simulink model "h175_model_stack_harness"  (R2023a)
settings: Solver=VariableStepAuto  StartTime=0.0  StopTime=4750  MaxStep=50  RelTol=1e-2
undefined symbols (not defined in the file): N2_T, sigbuilder_block
libraries: fl_lib x13, nesl_utility x11, SimscapeFluids_lib x2
(part 1 of 3)
settings Model: Creator=adrian.taveras  LastModifiedBy=stefan.notter
settings SolverCC: MaxConsecutiveMinStep=10  DecoupledContinuousIntegration=on
settings SimscapeCC: SimscapeLogType=all

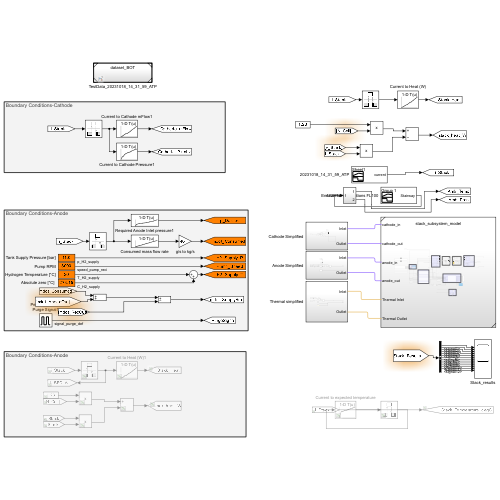
[thumbnail: Simulink's stored preview of the top-level diagram]
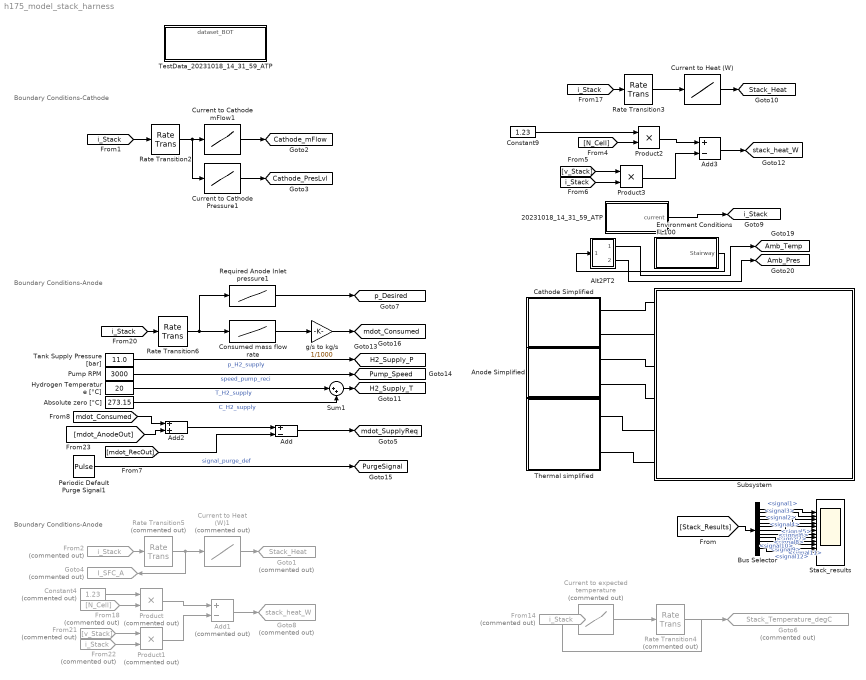
== system h175_model_stack_harness ==
  note: Boundary Conditions-Cathode
  note: Boundary Conditions-Anode
  note: Boundary Conditions-Anode
  20231018_14_31_59_ATP : Subsystem  Tag=STV Subsys  LoadFcn=sigbuilder_block('load');  StartFcn=sigbuilder_block('start');  StopFcn=sigbuilder_block('stop');  ClipboardFcn=sigbuilder_block('clipboard');  mask(Sigbuilder block){tuvar=[0:10]}
      mask help: Simulink:masks:SigbuilderBlock_MD
      mask init:
      | if ~strcmp(get_param(bdroot(gcbh),'SimulationStatus'),'stopped') tuvar = sigbuilder_block('maskInit'); end
      settings: CopyFcn=sigbuilder_block('copy');  DeleteFcn=sigbuilder_block('delete');  ModelCloseFcn=sigbuilder_block('modelClose');  PreSaveFcn=sigbuilder_block('preSave');  PauseFcn=sigbuilder_block('pause');  ContinueFcn=sigbuilder_block('continue');  NameChangeFcn=sigbuilder_block('namechange');  OpenFcn=sigbuilder_block('open',[725.25 330.75 938.25 556.5 ]);  CloseFcn=sigbuilder_block('close');
      mask Display: plot(0, 0, 100, 100,[2, 2, 32, 32, 2], [68, 8, 8, 68, 68],[32, 2], [38, 38], [32, 19, 2],[53, 60, 44], [32, 17, 17, 2],[16, 16, 31, 31]);txt = getActiveGroup(gcbh);text(2, 100, txt,'verticalAlignment', 'top');
  "Absolute zero [°C] " : Constant  Value=273.15
  Add : Sum  Inputs=+-
  Add1 : Sum  Commented=on  Inputs=+-
  Add2 : Sum
  Add3 : Sum  Inputs=+-
  Alt2PT2 : Subsystem
  Anode Simplified : Subsystem
  Bus Selector : BusSelector  OutputSignals=signal1,signal2,signal3,signal4,signal5,signal6,signal7,signal8,signal9,signal10,signal11,signal12
  Cathode Simplified : Subsystem
  Constant4 : Constant  Commented=on  Value=1.23
  Constant9 : Constant  Value=1.23
  Consumed mass flow rate : Lookup_n-D  NumberOfTableDimensions=1  BreakpointsForDimension1=[0;20;100;200;300;400;500;600]  Table=[0;0.1;0.5;1;1.5;2;2.5;3]  InternalRulePriority=Speed  RndMeth=Simplest
  Current to Cathode Pressure1 : Lookup_n-D  NumberOfTableDimensions=1  BreakpointsForDimension1=[0;50;100;150;200;250;300;350;400;510;600]  Table=[101330;140000;150000;175000;185000;195000;202500;210000;220000;235000;250000]  InternalRulePriority=Speed  RndMeth=Simplest
  Current to Cathode mFlow1 : Lookup_n-D  NumberOfTableDimensions=1  BreakpointsForDimension1=[0;50;100;150;200;250;300;350;400;510;600]  Table=[0;0.01;0.0225;0.035;0.045;0.055;0.068;0.0825;0.1;0.135;0.167]  InternalRulePriority=Speed  RndMeth=Simplest
  Current to Heat (W) : Lookup_n-D  NumberOfTableDimensions=1  BreakpointsForDimension1=[0:50:400]  Table=[0, 9932, 21438, 33442,47123, 59491, 77033, 93585, 112042]  InternalRulePriority=Speed  RndMeth=Simplest
  Current to Heat (W)1 : Lookup_n-D  Commented=on  NumberOfTableDimensions=1  BreakpointsForDimension1=[0:50:400]  Table=[0, 9932, 21438, 33442,47123, 59491, 77033, 93585, 112042]  InternalRulePriority=Speed  RndMeth=Simplest
  Current to expected temperature : Lookup_n-D  Commented=on  NumberOfTableDimensions=1  BreakpointsForDimension1=[0 50 100 150 200 250 300 350 400]  Table=[60 78 80 82 84 86 88 90 93]  InternalRulePriority=Speed  RndMeth=Simplest
  Environment Conditions FL100 : Subsystem  Tag=STV Subsys  LoadFcn=sigbuilder_block('load');  StartFcn=sigbuilder_block('start');  StopFcn=sigbuilder_block('stop');  ClipboardFcn=sigbuilder_block('clipboard');  mask(Sigbuilder block){tuvar=[0:10]}
      mask help: Simulink:masks:SigbuilderBlock_MD
      mask init:
      | if ~strcmp(get_param(bdroot(gcbh),'SimulationStatus'),'stopped') tuvar = sigbuilder_block('maskInit'); end
      settings: CopyFcn=sigbuilder_block('copy');  DeleteFcn=sigbuilder_block('delete');  ModelCloseFcn=sigbuilder_block('modelClose');  PreSaveFcn=sigbuilder_block('preSave');  PauseFcn=sigbuilder_block('pause');  ContinueFcn=sigbuilder_block('continue');  NameChangeFcn=sigbuilder_block('namechange');  OpenFcn=sigbuilder_block('open',[6 30 1908 951.75 ]);  CloseFcn=sigbuilder_block('close');
      mask Display: plot(0, 0, 100, 100,[2, 2, 32, 32, 2], [68, 8, 8, 68, 68],[32, 2], [38, 38], [32, 19, 2],[53, 60, 44], [32, 17, 17, 2],[16, 16, 31, 31]);txt = getActiveGroup(gcbh);text(2, 100, txt,'verticalAlignment', 'top');
  From14 : From  Commented=on  GotoTag=i_Stack  TagVisibility=global
  From18 : From  Commented=on  GotoTag=N_Cell
  From2 : From  Commented=on  GotoTag=i_Stack  TagVisibility=global
  From21 : From  Commented=on  GotoTag=v_Stack  TagVisibility=global
  From22 : From  Commented=on  GotoTag=i_Stack  TagVisibility=global
  Goto1 : Goto  Commented=on  GotoTag=Stack_Heat  TagVisibility=global
  Goto4 : Goto  Commented=on  GotoTag=I_SFC_A  TagVisibility=global
  Goto6 : Goto  Commented=on  GotoTag=Stack_Temperature_degC  TagVisibility=global
  Goto8 : Goto  Commented=on  GotoTag=stack_heat_W  TagVisibility=global
  Hydrogen Temperature [°C] : Constant  Value=20
  Periodic Default Purge Signal1 : DiscretePulseGenerator  PulseType=Time based  Period=3  PulseWidth=5
  Product : Product  Commented=on
  Product1 : Product  Commented=on
  Product2 : Product
  Product3 : Product
  Pump RPM : Constant  Value=3000
  Rate Transition2 : RateTransition
  Rate Transition3 : RateTransition
  Rate Transition4 : RateTransition  Commented=on
  Rate Transition5 : RateTransition  Commented=on
  Rate Transition6 : RateTransition
  Required Anode Inlet pressure1 : Lookup_n-D  NumberOfTableDimensions=1  BreakpointsForDimension1=[0;20;100;200;300;400;500;600]  Table=[1;1.4;1.6;1.7;1.8;2;2.3;2.6]  InternalRulePriority=Speed  RndMeth=Simplest
  Stack_results : Scope  NumInputPorts=12
  Subsystem : Subsystem  InitFcn=|  ReferencedSubsystem=stack_subsystem_model
      | addpath(genpath('p10_doe_files/'))
      | run('stack_subsystem_parameters.m')
      | run('stack_subsystem_supply_bus_definitions.m')
      settings: PortSchema="{\"entries\":[{\"content\":{\"sides\":[{\"content\":{\"connectorIds\":[\"RConn1\",\"RConn2\",\"LConn1\",\"LConn2\",\"LConn3\",\"LConn4\"]},\"type\":\"ConnectorPlacement.EquallySpacedRectSide\",\"uuid\":\"f7417d0d-e48e-4edc-84f7-16cb6b1fd341\"},{\"content\":{\"side\":\"RIGHT\"},\"type\":\"ConnectorPlacement.EquallySpacedRectSide\",\"uuid\":\"dd727874-0c87-4720-9a58-e9e43c2cfc5b\"},{\"content\":{\"side\":\"TOP\"},\"type\":\"ConnectorPlacement.EquallySpacedRectSide\",\"uuid\":\"042cb514-9034-4c64-aaa6-55fccd9e3c82\"},{\"content\":{\"side\":\"BOTTOM\"},\"type\":\"ConnectorPlacement.EquallySpacedRectSide\",\"uuid\":\"dba865e7-7c98-4866-84bd-6f3d01b8a3bd\"}]},\"type\":\"ConnectorPlacement.EquallySpacedConnector\",\"uuid\":\"b4ac4c8a-745a-415f-9259-8b2ea3c16805\"}],\"packageUris\":[\"http://schema.mathworks.com/mf0/Connector/R2020b\"],\"version\":\"1.0\"}"
  Sum1 : Sum  Inputs=|++
  Tank Supply Pressure [bar] : Constant  Value=11.0
  TestData_20231018_14_31_59_ATP : ModelReference  ModelNameDialog=dataset_BOT.slx  SimulationMode=Normal  ModelReferenceVersion=1.3
  Thermal simplified : Subsystem
  g/s to kg/s : Gain  Gain=1/1000
  tag scope: Amb_Pres=global, Amb_Temp=global, Cathode_PresLvl=global, Cathode_mFlow=global, H2_Supply_P=global, H2_Supply_T=global, Pump_Speed=global, PurgeSignal=global, Stack_Heat=global, i_Stack=global, mdot_Consumed=global, mdot_SupplyReq=global, p_Desired=global, stack_heat_W=global
  wires:
  [mdot_RecOut] -> Add/2
  [mdot_AnodeOut] -> Add2/2
  Add2/1 -> Add/1
  Product1/1 -> Add1/2
  Rate Transition4/1 -> Current to expected temperature/1
  Required Anode Inlet pressure1/1 -> [p_Desired]
  [i_Stack] -> Rate Transition2/1
  From14/1 -> Rate Transition4/1
  Current to Cathode Pressure1/1 -> [Cathode_PresLvl]
  Constant4/1 -> Product/1
  [mdot_Consumed] -> Add2/1
  Periodic Default Purge Signal1/1 -> [PurgeSignal]  "signal_purge_def"
  From18/1 -> Product/2
  Product/1 -> Add1/1
  Add1/1 -> Goto8/1
  From22/1 -> Product1/2
  Current to Heat (W)1/1 -> Goto1/1
  Current to Cathode mFlow1/1 -> [Cathode_mFlow]
  [i_Stack] -> Rate Transition6/1
  From2/1 -> Rate Transition5/1
  Current to expected temperature/1 -> Goto6/1
  Rate Transition6/1 -> Required Anode Inlet pressure1/1, Consumed mass flow rate/1
  Rate Transition2/1 -> Current to Cathode Pressure1/1, Current to Cathode mFlow1/1
  Rate Transition5/1 -> Goto4/1, Current to Heat (W)1/1
  Tank Supply Pressure [bar]/1 -> [H2_Supply_P]  "p_H2_supply"
  Pump RPM/1 -> [Pump_Speed]  "speed_pump_reci"
  From21/1 -> Product1/1
  Add/1 -> [mdot_SupplyReq]
  Hydrogen Temperature [°C]/1 -> Sum1/1  "T_H2_supply"
  "Absolute zero [°C] "/1 -> Sum1/2  "C_H2_supply"
  g/s to kg/s/1 -> [mdot_Consumed]
  Sum1/1 -> [H2_Supply_T]
  Consumed mass flow rate/1 -> g/s to kg/s/1
  Alt2PT2/2(Out2) -> [Amb_Pres]
  Environment Conditions FL100/1(Stairway) -> Alt2PT2/1(In1)
  Alt2PT2/1(Out1) -> [Amb_Temp]
  Product3/1 -> Add3/2
  [v_Stack] -> Product3/1
  Constant9/1 -> Product2/1
  Product2/1 -> Add3/1
  [i_Stack] -> Product3/2
  Add3/1 -> [stack_heat_W]
  Current to Heat (W)/1 -> [Stack_Heat]
  [i_Stack] -> Rate Transition3/1
  Rate Transition3/1 -> Current to Heat (W)/1
  [N_Cell] -> Product2/2
  20231018_14_31_59_ATP/1(current) -> [i_Stack]
  [Stack_Results] -> Bus Selector/1
  Bus Selector/1 -> Stack_results/1  "<signal1>"
  Bus Selector/2 -> Stack_results/2  "<signal2>"
  Bus Selector/3 -> Stack_results/3  "<signal3>"
  Bus Selector/4 -> Stack_results/4  "<signal4>"
  Bus Selector/5 -> Stack_results/5  "<signal5>"
  Bus Selector/6 -> Stack_results/6  "<signal6>"
  Bus Selector/7 -> Stack_results/7  "<signal7>"
  Bus Selector/8 -> Stack_results/8  "<signal8>"
  Bus Selector/9 -> Stack_results/10  "<signal9>"
  Bus Selector/10 -> Stack_results/9  "<signal10>"
  Bus Selector/11 -> Stack_results/11  "<signal11>"
  Bus Selector/12 -> Stack_results/12  "<signal12>"
  connections:
  Thermal simplified/RConn1 -- Subsystem/LConn3
  Subsystem/LConn4 -- Thermal simplified/RConn2
  Anode Simplified/RConn1 -- Subsystem/LConn1
  Anode Simplified/RConn2 -- Subsystem/LConn2
  Cathode Simplified/RConn1 -- Subsystem/RConn1
  Cathode Simplified/RConn2 -- Subsystem/RConn2

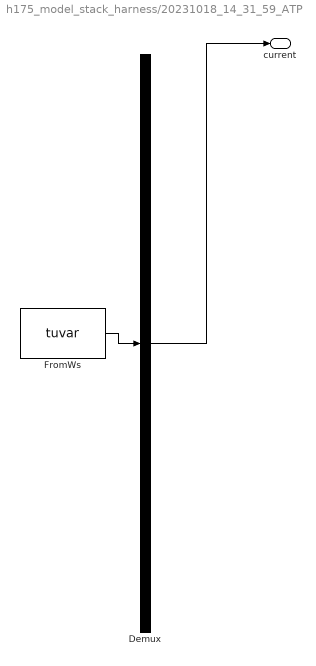
== system h175_model_stack_harness/20231018_14_31_59_ATP ==
  Demux : Demux  Tag=STV Demux  Outputs=1
      settings: DisplayOption=none
  FromWs : FromWorkspace  Tag=STV FromWs  VariableName=tuvar
      SigBuilderData=|
      | common.afterFinalStr = 'Extrapolate'
      | common.sampleTime = 0
      | dataSet.timeRange = [0 4735]
      | dataSet.name = 'Sheet1'
      | sbobj.Groups.Name = 'Sheet1'
      | sbobj.Groups.Signals.Name = 'current'
      | sbobj.Groups.Signals.XData = [0 710 730 830 850 1000 1020 1080 1100 1200 1230 1260 1270 1320 1340 1390 1405 1455 1475 1525 1565 3990 4000 4030 4090 4130 4245 4270 4345 4355 4385 4395 4735]
      | sbobj.Groups.Signals.YData = [5 5 45 45 100 100 200 200 300 300 45 45 50 50 200 200 300 300 100 100 420 420 340 420 260 340 340 50 50 45 45 5 5]
      | sbobj.Groups.TimeRange = [0 4735]
  current : Outport  Tag=STV Outport
  wires:
  Demux/1 -> current/1
  FromWs/1 -> Demux/1

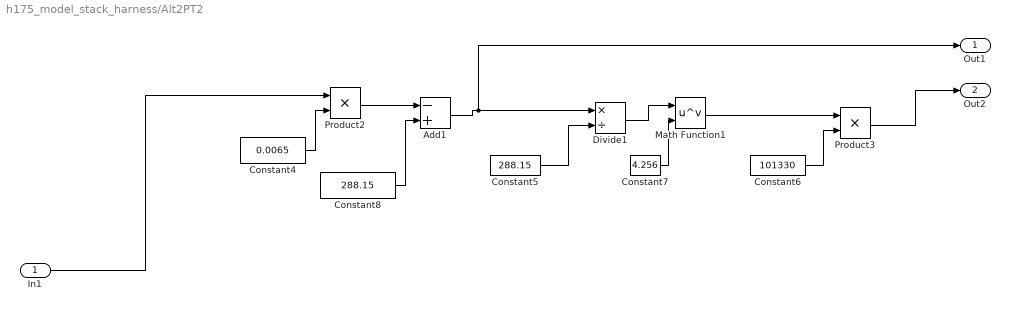
== system h175_model_stack_harness/Alt2PT2 ==
  In1 : Inport
  Add1 : Sum  Inputs=-+
  Constant4 : Constant  Value=0.0065
  Constant5 : Constant  Value=288.15
  Constant6 : Constant  Value=101330
  Constant7 : Constant  Value=4.256
  Constant8 : Constant  Value=288.15
  Divide1 : Product  Inputs=*/
  Math Function1 : Math  Operator=pow
  Product2 : Product
  Product3 : Product
  Out1 : Outport
  Out2 : Outport  Port=2
  wires:
  Constant5/1 -> Divide1/2
  Constant8/1 -> Add1/2
  In1/1 -> Product2/1
  Add1/1 -> Out1/1, Divide1/1
  Constant4/1 -> Product2/2
  Math Function1/1 -> Product3/1
  Constant7/1 -> Math Function1/2
  Divide1/1 -> Math Function1/1
  Product2/1 -> Add1/1
  Constant6/1 -> Product3/2
  Product3/1 -> Out2/1

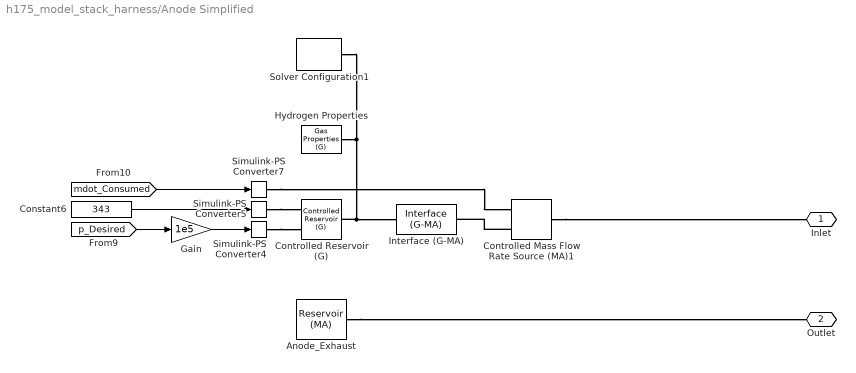
== system h175_model_stack_harness/Anode Simplified ==
  Anode_Exhaust : fl_lib/Moist Air/Elements/Reservoir (MA)  pressure_spec=foundation.enum.pressure_spec.specified  reservoir_pressure=2 bar  temperature_spec=foundation.enum.temperature_spec.specified  reservoir_temperature=95 degC  moisture_spec=foundation.enum.moistureSpec.RelativeHumidity  reservoir_RH=0.68  reservoir_x_w=0.01  reservoir_y_w=0.01  reservoir_HR=0.01  reservoir_Tw=287 K  trace_gas_spec=foundation.enum.trace_gas_spec.mass_fraction  reservoir_x_g=0.001  reservoir_y_g=0.001  RH_ws=1  area_A=0.01 m^2
  Constant6 : Constant  Value=343
  Controlled Mass Flow Rate Source (MA)1 : fl_lib/Moist Air/Sources/Controlled Mass Flow Rate Source (MA)  power_spec=foundation.enum.power_spec.none  area_A=0.00358 m^2  area_B=0.00358 m^2
      settings: InternalSimscapePortConfiguration="{\"Bottom\":[],\"Left\":[{\"id\":\"A\",\"label\":\"A\",\"type\":\"foundation.moist_air.moist_air\"},{\"id\":\"M\",\"label\":\"M\",\"type\":\"input\"}],\"Right\":[{\"id\":\"B\",\"label\":\"B\",\"type\":\"foundation.moist_air.moist_air\"}],\"Top\":[]}"
  Controlled Reservoir (G) : fl_lib/Gas/Elements/Controlled Reservoir (G)  area_A=0.00358 m^2
      settings: InternalSimscapePortConfiguration="{\"Bottom\":[],\"Left\":[{\"id\":\"A\",\"label\":\"A\",\"type\":\"foundation.gas.gas\"}],\"Right\":[{\"id\":\"T_in\",\"label\":\"T\",\"type\":\"input\"},{\"id\":\"p_in\",\"label\":\"P\",\"type\":\"input\"}],\"Top\":[]}"
  Gain : Gain  Gain=1e5
  Hydrogen Properties : fl_lib/Gas/Utilities/Gas Properties (G)  gas_spec=foundation.enum.gas_spec.real_gas  R=0.287 kJ/(K*kg)  Z=1  T_ref=293.15 K  h_ref=420 kJ/kg  cp_ref=1 kJ/(K*kg)  mu_ref=18 s*uPa  k_ref=26 mW/(K*m)  T_TLU1=[150 : 10 : 200, 250 : 50 : 1000, 1500, 2000]' K  h_TLU1=[275.264783730547; 285.377054177734; 295.474578903607; 305.560871069627; 315.638490783961; 325.709373787179; 376.008033649461; 426.297784741196; 476.678788323875; 527.253890684429; 578.12722735187; 629.395040865183; 681.137690131207; 733.415442873049; 786.267894376777; 839.715851152006; 893.764459999509; 948.406676876931; 1003.62653219711; 1059.40193232821; 1115.70691941005; 1172.51341226958; 1762.18512007361; 2377.14064127409] kJ/kg  cp_TLU1=[1.01211492398124; 1.01042105529234; 1.00914159006373; 1.00815898273273; 1.00739688341918; 1.00680484569075; 1.00554191216852; 1.00637389921747; 1.0092105862442; 1.01414404435034; 1.02111299587909; 1.02986878923959; 1.04003820504128; 1.05120320041448; 1.06296312852444; 1.07497111709439; 1.08694865668905; 1.0986858495625; 1.11003396604319; 1.12089493621399; 1.13121051694521; 1.14095251451866; 1.21001953144; 1.24628356718428] kJ/(K*kg)  mu_TLU1=[10.3766056544352; 10.9908682444892; 11.5932000841352; 12.1841060353213; 12.764067709023; 13.3335437107148; 16.038149065057; 18.5373404836509; 20.8671495114253; 23.0554226800681; 25.1239717991959; 27.0901379793485; 28.96790749834; 30.7687111230031; 32.5020036481173; 34.17569027566; 35.7964450415303; 37.3699520751368; 38.9010908824946; 40.3940804368247; 41.8525925389218; 43.279841956487; 56.3254722619962; 68.068290080945] s*uPa  k_TLU1=[14.1517155766309; 15.0474512994325; 15.9300520513026; 16.7998749295306; 17.6573089963228; 18.5027588910197; 22.5644026699512; 26.384465676638; 30.0032801168886; 33.4532006033488; 36.7600619429332; 39.9446251241844; 43.0237448740114; 46.0112537033799; 48.9186234516389; 51.7554617696538; 54.5298878921773; 57.2488200454925; 59.9181976996146; 62.5431553064749; 65.128159527924; 67.6771186900213; 91.7815514375552; 114.486299090693] mW/(K*m)  T_TLU2=H2.T K  p_TLU2=H2.p MPa  rho_TLU2=H2.rho kg/m^3  s_TLU2=H2.s kJ/(K*kg)  h_TLU2=H2.h kJ/kg  cp_TLU2=H2.cp kJ/(K*kg)  mu_TLU2=H2.mu s*uPa  k_TLU2=H2.k mW/(K*m)  beta_TLU2=H2.beta MPa  alpha_TLU2=H2.alpha 1/K  T_min_perfect=1 K  T_max_perfect=inf K  p_min_perfect=1 Pa  p_max_perfect=inf MPa  T_range_flag=foundation.enum.T_range_G.from_props  T_min_semiperfect=150 K  T_max_semiperfect=2000 K  p_min_semiperfect=1 Pa  p_max_semiperfect=inf MPa  pT_region_flag=foundation.enum.pT_region_G.from_props  pT_validity_TLU2=ones(24, 20)  T_min_real=150 K  T_max_real=2000 K  p_min_real=0.001 MPa  p_max_real=10 MPa  p_atm=0.101325 MPa  properties_range_check=simscape.enum.assert.action.error  Mach_rev=0.001 / 10
  Interface (G-MA) : SimscapeFluids_lib/Fluid Network Interfaces/Interface (G-MA)  interface_type=foundation.enum.constant_controlled.constant  moisture_spec=foundation.enum.moistureSpec.RelativeHumidity  RH_interface=0.0005  x_w_interface=0.01  y_w_interface=0.01  HR_interface=0.01  Tw_interface=287 K  trace_gas_spec=foundation.enum.trace_gas_spec.mass_fraction  x_g_interface=0.001  y_g_interface=0.001  RH_ws=1  area=0.00358 m^2  input_error_spec=foundation.enum.input_range_error.warn
      settings: InternalSimscapePortConfiguration="{\"Bottom\":[],\"Left\":[{\"id\":\"G\",\"label\":\"G\",\"type\":\"foundation.gas.gas\"}],\"Right\":[{\"id\":\"MA\",\"label\":\"MA\",\"type\":\"foundation.moist_air.moist_air\"}],\"Top\":[]}"
  Simulink-PS Converter4 : nesl_utility/Simulink-PS Converter  PhysicalDomain=network_engine_domain  SubClassName=ps_input  LeftPortType=input  RightPortType=output  PseudoPeriodic=off  Frequencies=[]  NoiseDistribution=none  NoiseParameters=[]  Unit=1  AffineConversion=off  FilteringAndDerivatives=provide  SimscapeFilterOrder=1  InputFilterTimeConstant=0.001  UdotUserProvided=0
  Simulink-PS Converter5 : nesl_utility/Simulink-PS Converter  PhysicalDomain=network_engine_domain  SubClassName=ps_input  LeftPortType=input  RightPortType=output  PseudoPeriodic=off  Frequencies=[]  NoiseDistribution=none  NoiseParameters=[]  Unit=1  AffineConversion=off  FilteringAndDerivatives=provide  SimscapeFilterOrder=1  InputFilterTimeConstant=0.001  UdotUserProvided=0
  Simulink-PS Converter7 : nesl_utility/Simulink-PS Converter  PhysicalDomain=network_engine_domain  SubClassName=ps_input  LeftPortType=input  RightPortType=output  PseudoPeriodic=off  Frequencies=[]  NoiseDistribution=none  NoiseParameters=[]  Unit=1  AffineConversion=off  FilteringAndDerivatives=provide  SimscapeFilterOrder=1  InputFilterTimeConstant=0.001  UdotUserProvided=0
  Solver Configuration1 : nesl_utility/Solver Configuration  PhysicalDomain=network_engine_domain  SubClassName=solver  LeftPortType=input  RightPortType=generic  Tones=[]  Harmonics=[]  SimulateNoise=off  Profile=off  UseLocalSampling=off  EnableSwitchedLinearOptims=on  FrequencyDomain=off  UseCCode=off  RelTol=0.001  AbsTol=0.001  MinStep=1e-09  ToWorkspace=off  RevertToSquareIcSolve=off  NumHomotopyIterations=100  PhasorMode=off  PhasorModeNumHarmonics=1  ConsistencySolver=NEWTON_XTOL_AFTER_FTOL  IndexReductionMethod=DerivativeReplacement  DoDC=off  ResidualTolerance=1e-09  ConsistencyTolSource=GLOBAL  ConsistencyAbsTol=0.001  ConsistencyRelTol=0.001  ConsistencyTolFactor=0.001  UseLocalSolver=off  LocalSolverChoice=NE_BACKWARD_EULER_ADVANCER  ResolveIndetEquations=on  FunctionEvalNumThread=1  LocalSolverSampleTime=0.001  DoFixedCost=off  MaxNonlinIter=3  MaxModeIter=2  ComputeImpulses=off  ImpulseIterations=2  LinearAlgebra=auto  LinearAlgebraNumThread=0  EquationFormulation=NE_TIME_EF  DelaysMemoryBudget=1024  AutomaticFiltering=on  FilteringTimeConstant=0.001  PartitionStorageMethod=AS_NEEDED  PartitionMemoryBudget=1024  PartitionMethod=ROBUST
  Inlet : PMIOPort  Side=Right
  Outlet : PMIOPort  Port=2  Side=Right
  wires:
  Constant6/1 -> Simulink-PS Converter5/1
  [p_Desired] -> Gain/1
  [mdot_Consumed] -> Simulink-PS Converter7/1
  Gain/1 -> Simulink-PS Converter4/1
  connections:
  Hydrogen Properties/RConn1 -- Interface (G-MA)/LConn1 -- Controlled Reservoir (G)/LConn1 -- Solver Configuration1/RConn1
  Simulink-PS Converter4/RConn1 -- Controlled Reservoir (G)/RConn2
  Controlled Mass Flow Rate Source (MA)1/LConn1 -- Interface (G-MA)/RConn1
  Simulink-PS Converter7/RConn1 -- Controlled Mass Flow Rate Source (MA)1/LConn2
  Simulink-PS Converter5/RConn1 -- Controlled Reservoir (G)/RConn1
  Anode_Exhaust/LConn1 -- Outlet/RConn1
  Controlled Mass Flow Rate Source (MA)1/RConn1 -- Inlet/RConn1
